simulink model "Lab3"  (R2014b)
settings: Solver=FixedStepDiscrete  StartTime=0.0  StopTime=100  FixedStep=.001  RelTol=1e-3
libraries: embdlinuxlib x3, dspswit3 x1, dspsigops x1
settings Model: SimulationMode=external  ExtModeTrigDuration=100  Creator=Becky  LastModifiedBy=rreck
settings OptimizationCC: OptimizeModelRefInitCode=on  LifeSpan=1
settings DebuggingCC: UnderspecifiedInitializationDetection=Classic  MergeDetectMultiDrivingBlocksExec=none  SolverPrmCheckMsg=none
settings HardwareCC: ProdLargestAtomicInteger=Long  ProdLargestAtomicFloat=Double  ProdEndianess=LittleEndian  ProdHWDeviceType=ARM Compatible->ARM Cortex
settings RTWCC: SystemTargetFile=realtime.tlc  GenerateMakefile=off  TemplateMakefile=realtime.tmf  Description=Run on Target Hardware  RTWVerbose=off  ProcessScript=realtime_make_rtw_hook
settings STFCustomTargetCC: TargetLibSuffix=.a  GenerateSampleERTMain=on  ERTCustomFileBanners=on  SupportNonInlinedSFcns=off  SupportVariableSizeSignals=on  MATLABClassNameForMDSCustomization=Simulink.SoftwareTarget.ERTCustomization  GRTInterface=off  SystemTargetFile=realtime.tlc
settings ERTTargetCC: GenerateSampleERTMain=on  ParMdlRefBuildCompliant=off  CompOptLevelCompliant=off  ConcurrentExecutionCompliant=off  CombineOutputUpdateFcns=off  ERTFirstTimeCompliant=off  SupportContinuousTime=on  SupportVariableSizeSignals=on  ModelStepFunctionPrototypeControlCompliant=off  CPPClassGenCompliant=off  ExtModeMexArgs='192.168.0.3' 0 17725  InlinedParameterPlacement=NonHierarchical  ERTSrcFileBannerTemplate=realtime_code_template.cgt  ERTHdrFileBannerTemplate=realtime_code_template.cgt  ERTDataSrcFileTemplate=realtime_code_template.cgt  ERTDataHdrFileTemplate=realtime_code_template.cgt  ERTCustomFileTemplate=realtime_file_process.tlc

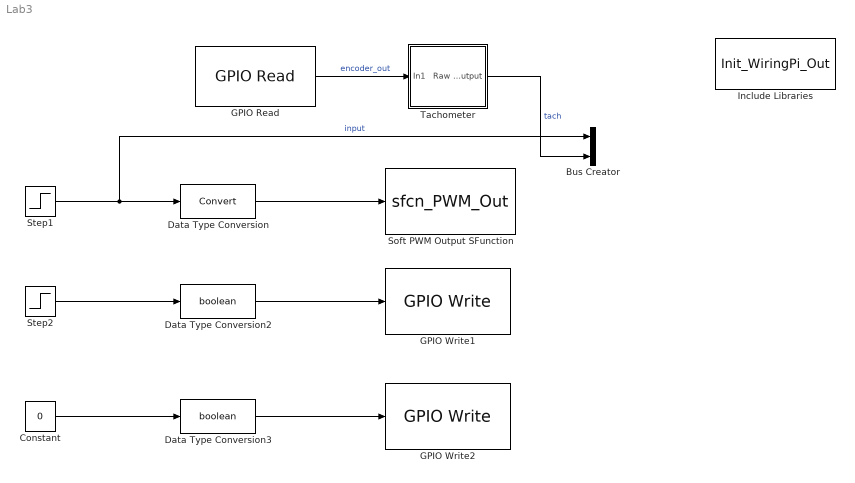
== system Lab3 ==
  Bus Creator : BusCreator  Inputs=2
  Constant : Constant  Value=0
  Data Type Conversion : DataTypeConversion
  Data Type Conversion2 : DataTypeConversion  OutDataTypeStr=boolean
  Data Type Conversion3 : DataTypeConversion  OutDataTypeStr=boolean
  GPIO Read : embdlinuxlib/GPIO Read  board=Model B Rev2  gpio=22  internalResistor=Off  sampleTime=0.001  direction=Input  blockPlatform=Raspberry Pi
  GPIO Write1 : embdlinuxlib/GPIO Write  board=Model B Rev2  gpio=18  direction=Output  blockPlatform=Raspberry Pi
  GPIO Write2 : embdlinuxlib/GPIO Write  board=Model B Rev2  gpio=4  direction=Output  blockPlatform=Raspberry Pi
  Include Libraries : S-Function  InitFcn=try, set_param(gcb,'FunctionName','Init_WiringPi_Out'), end  FunctionName=Init_WiringPi_Out  Parameters=uint8(0),uint8(7)  SFunctionModules=Init_WiringPi_Out_wrapper  EnableBusSupport=off  mask(S-Function Builder){}
      mask init:
      | val = [[.9  0.75 0.75 1 1 .9 .9 1]',[1 1 0.75 0.75 .9 .9 1 .9]'];try , sys = get_param(gcb,'SfunBuilderFcnName');if isempty(sys), sys = get_param(gcb,'FunctionName'); end,catch, sys = get_param(gcb,'FunctionName'); end
      settings: CopyFcn=set_param(gcbh,'LinkStatus','none')  PreSaveFcn=try, set_param(gcb,'FunctionName','Init_WiringPi_Out'), end  OpenFcn=sfunctionwizard(gcbh)
      mask Display: plot(val(:,1),val(:,2)),disp(sys)
  Soft PWM Output SFunction : S-Function  InitFcn=try, set_param(gcb,'FunctionName','sfcn_PWM_Out'), end  FunctionName=sfcn_PWM_Out  Parameters=uint8(0)  SFunctionModules=sfcn_PWM_Out_wrapper  EnableBusSupport=off  mask(S-Function Builder){}
      mask init: same as Lab3/Include Libraries
      settings: CopyFcn=set_param(gcbh,'LinkStatus','none')  PreSaveFcn=try, set_param(gcb,'FunctionName','sfcn_PWM_Out'), end  OpenFcn=sfunctionwizard(gcbh)
      mask Display: plot(val(:,1),val(:,2)),disp(sys), port_label('input',1,'in')
  Step1 : Step  Time=2  Before=25  After=75  SampleTime=0
  Step2 : Step  Time=99.5  Before=1  After=0  SampleTime=0
  Tachometer : Subsystem
  wires:
  GPIO Read/1 -> Tachometer/1(In1)  "encoder_out"
  Data Type Conversion2/1 -> GPIO Write1/1
  Step2/1 -> Data Type Conversion2/1
  Constant/1 -> Data Type Conversion3/1
  Data Type Conversion3/1 -> GPIO Write2/1
  Step1/1 -> Bus Creator/1, Data Type Conversion/1  "input"
  Data Type Conversion/1 -> Soft PWM Output SFunction/1
  Tachometer/1(Raw Output) -> Bus Creator/2  "tach"

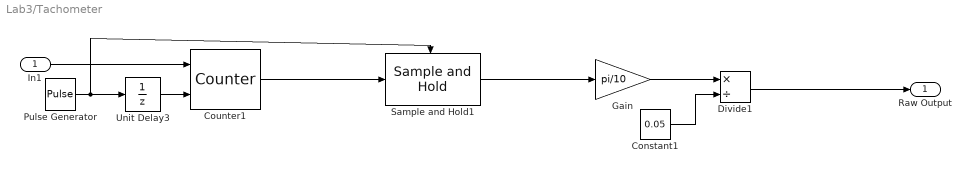
== system Lab3/Tachometer ==
  In1 : Inport
  Constant1 : Constant  Value=0.05
  Counter1 : dspswit3/Counter  Direction=Up  CountEvent=Rising edge  CounterSize=User defined  MaxCount=256  InitialCount=0  Output=Count  HitValue=1  ResetInput=on  SamplesPerFrame=1  Ts=1  CntDtype=double  HitDtype=Logical
  Divide1 : Product  Inputs=*/
  Gain : Gain  Gain=pi/10
  Pulse Generator : DiscretePulseGenerator  PulseType=Time based  Period=.05  PulseWidth=10
  Sample and Hold1 : dspsigops/Sample and Hold  trig=Rising edge  initCond=1  latchinput=off
  Unit Delay3 : UnitDelay  SampleTime=-1
  Raw Output : Outport
  wires:
  In1/1 -> Counter1/1
  Counter1/1 -> Sample and Hold1/1
  Constant1/1 -> Divide1/2
  Divide1/1 -> Raw Output/1
  Pulse Generator/1 -> Sample and Hold1/Trigger, Unit Delay3/1
  Gain/1 -> Divide1/1
  Unit Delay3/1 -> Counter1/2
  Sample and Hold1/1 -> Gain/1
